simulink model "OSWEC_w_Mechanical_PTO"  (R2014b)
settings: Solver=ode4  StartTime=0  StopTime=400  FixedStep=0.001  RelTol=1e-3
values from neighbouring files (symbols this model uses):
  ptosim = ptoSimClass('Direct Drive Linear Generator')    [ptoSimInputFile.m]
undefined symbols (not defined in the file or in its folder): body, constraint, pto
libraries: WECSim_Lib x5, PTOSim_Lib x2
settings Model: Creator=mlawson  LastModifiedBy=rso
settings SolverCC: AlgebraicLoopSolver=LineSearch
settings DataIOCC: LimitDataPoints=off  SaveOutput=off  SaveTime=off
settings DebuggingCC: UnderspecifiedInitializationDetection=Classic  MergeDetectMultiDrivingBlocksExec=none  StateNameClashWarn=warning
settings ExplorerConfigSet: InternalSimMechanicsExplorerSettings="<ExplorerConfiguration><canonicalview>default</canonicalview><TilePanel><TileInfo><Tiles Columns=\"1\" Count=\"1\" Rows=\"1\"><Column Left=\"2\" Weight=\"1\"/><Column Left=\"1335\"/><Row Top=\"2\" Weight=\"1\"/><Row Top=\"911\"/><Tile Height=\"1\" Width=\"1\" X=\"0\" Y=\"0\"/></Tiles></TileInfo><SceneInfo><SceneViewer><BGColor><R>0.60000002384185791</R><G>0.60000002384185791</G><B>0.60000002384185791</B></BGColor><Camera><Position><X>365.37645888990272</X><Y>-369.82486814446582</Y><Z>359.64809521743916</Z></Position><Center><X>-6.7351450971904585</X><Y>2.2867358426280204</Y><Z>-12.463508769654169</Z></Center><Up><X>-0.40824829046386307</X><Y>0.40824829046386307</Y><Z>0.81649658092772615</Z></Up><Left>-57.820127362122818</Left><Right>57.820127362122818</Right><Bottom>-38.308817187253304</Bottom><Top>38.308817187253304</Top></Camera></SceneViewer></SceneInfo></TilePanel></ExplorerConfiguration>"

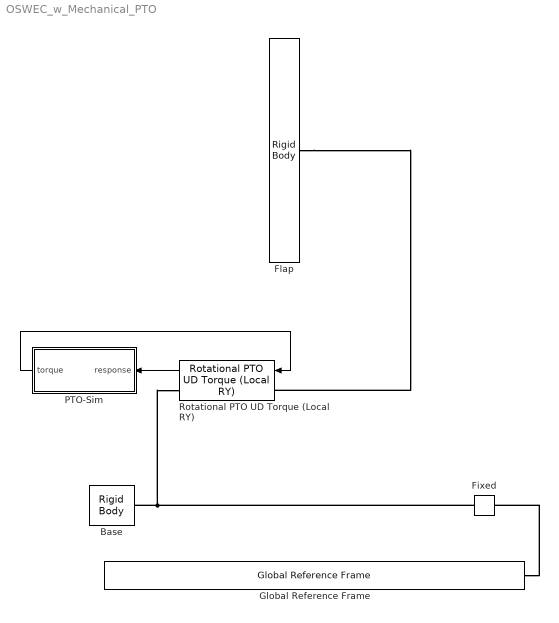
== system OSWEC_w_Mechanical_PTO ==
  Base : WECSim_Lib/Body Elements/Rigid Body  body=body(2)
      settings: AttributesFormatString=%<body>
  Fixed : WECSim_Lib/Constraints/Fixed  constraint=constraint(1)
      settings: AttributesFormatString=%<constraint>
  Flap : WECSim_Lib/Body Elements/Rigid Body  body=body(1)
      settings: AttributesFormatString=%<body>
  Global Reference Frame : WECSim_Lib/Frames/Global Reference Frame  waves=waves  simu=simu
  PTO-Sim : Subsystem
  Rotational PTO UD Torque (Local RY) : WECSim_Lib/PTOs/Rotational PTO UD Torque (Local RY)  pto=pto(1)
      settings: AttributesFormatString=%<pto>
  wires:
  Rotational PTO UD Torque (Local RY)/1 -> PTO-Sim/1(response)
  PTO-Sim/1(torque) -> Rotational PTO UD Torque (Local RY)/1
  connections:
  Global Reference Frame/RConn1 -- Fixed/LConn1
  Fixed/RConn1 -- Rotational PTO UD Torque (Local RY)/RConn1 -- Base/RConn1
  Flap/RConn1 -- Rotational PTO UD Torque (Local RY)/LConn1

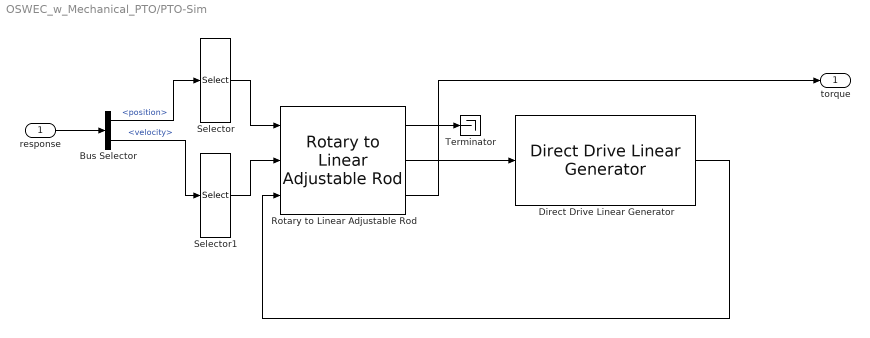
== system OSWEC_w_Mechanical_PTO/PTO-Sim ==
  response : Inport
  Bus Selector : BusSelector  OutputSignals=position,velocity
  Direct Drive Linear Generator : PTOSim_Lib/ Generator/Direct Drive Linear Generator  ptosim=ptosim.linearGenerator(1)
  Rotary to Linear Adjustable Rod : PTOSim_Lib/Motion Conversion/Rotary to Linear Adjustable Rod  ptosim=ptosim.motionMechanism
  Selector : Selector  InputPortWidth=6  Indices=5
  Selector1 : Selector  InputPortWidth=6  Indices=5
  Terminator : Terminator
  torque : Outport
  wires:
  response/1 -> Bus Selector/1
  Bus Selector/1 -> Selector/1  "<position>"
  Bus Selector/2 -> Selector1/1  "<velocity>"
  Rotary to Linear Adjustable Rod/3 -> torque/1
  Selector/1 -> Rotary to Linear Adjustable Rod/1
  Selector1/1 -> Rotary to Linear Adjustable Rod/2
  Rotary to Linear Adjustable Rod/2 -> Direct Drive Linear Generator/1
  Rotary to Linear Adjustable Rod/1 -> Terminator/1
  Direct Drive Linear Generator/1 -> Rotary to Linear Adjustable Rod/3
